simulink model "ap_12B_cocoSim_pp"  (Simulink 8.5)
settings: Solver=ode3  StartTime=0.0  StopTime=100  FixedStep=Ts  RelTol=1e-3
undefined symbols (not defined in the file): beaver_b, beaver_c, beaver_mass, beaver_S, Cl0, Cl_alpha2_dpt, Cl_beta, Cl_da, Cl_da_alpha, Cl_dr, Cl_p, Cl_r, Cm0, Cm_alpha, Cm_alpha2, Cm_beta2, Cm_de, Cm_df, Cm_dpt, Cm_q, Cm_r, Cn0, Cn_beta, Cn_beta3, Cn_da, Cn_dpt3, Cn_dr, Cn_p, Cn_q, Cn_r, Cx0, Cx_alpha, Cx_alpha2, Cx_alpha3, Cx_df, Cx_df_alpha, Cx_dpt, Cx_dpt2_alpha, Cx_dr, Cx_q, Cy0, Cy_beta, Cy_da, Cy_dr, Cy_dr_alpha, Cy_p, Cy_r, Cz0, Cz_alpha, Cz_alpha3, Cz_de, Cz_de_beta, Cz_df, Cz_df_alpha, Cz_dpt, Cz_q, d2r, fin_act_1, fin_act_2, fin_act_3 ... (+23)
libraries: simulink x12, aerolibtransform2 x9, aerolibutil x7, aerolibasang x7, aerolibadynsys x3, aerolib6dofsys x2, aerolib6dof2 x1
(part 2 of 3)

== system ap_12B_cocoSim_pp/Autopilot/Roll_Autopilot/Roll Reference ==
  note: Roll Reference
  Phi : Inport  RequirementInfo={'other' 'do178b_autopilot_requirements.docx' '@Simulink_requirement_item_3' 'true' '1.3. Roll Hold Reference' '' } %GIDa_7be110a1_1244_43c5_a751_2715cb6886db
  AP eng : Inport  RequirementInfo={'other' 'do178b_autopilot_requirements.docx' '@Simulink_requirement_item_3' 'true' '1.3. Roll Hold Reference' '' } %GIDa_7321b38e_2b45_4502_bb86_556b63306af0  Port=2
  Turn Knob : Inport  RequirementInfo={'other' 'do178b_autopilot_requirements.docx' '@Simulink_requirement_item_3' 'true' '1.3. Roll Hold Reference' '' } %GIDa_fd11246b_c871_46a3_9662_7459fa475b84  Port=3
  Abs : Abs  RequirementInfo={'other' 'do178b_autopilot_requirements.docx' '@Simulink_requirement_item_3' 'true' '1.3. Roll Hold Reference' '' } %GIDa_7c5a478a_1c5c_492b_92bb_3b8cbe69ec92
  Not engaged : Logic  RequirementInfo={'other' 'do178b_autopilot_requirements.docx' '@Simulink_requirement_item_3' 'true' '1.3. Roll Hold Reference' '' } %GIDa_f8de7ddf_282c_452d_ba2b_b5d1c603b30d  Operator=NOT  IconShape=distinctive  AllPortsSameDT=off  OutDataTypeStr=boolean
  Ref Threshold : RelationalOperator  RequirementInfo={'other' 'do178b_autopilot_requirements.docx' '@Simulink_requirement_item_3' 'true' '1.3. Roll Hold Reference' '' } %GIDa_5bcc0fb3_b840_4e41_b948_77b94adee73e  OutDataTypeStr=boolean  InputSameDT=on
  Ref Threshold1 : RelationalOperator  RequirementInfo={'other' 'do178b_autopilot_requirements.docx' '@Simulink_requirement_item_3' 'true' '1.3. Roll Hold Reference' '' } %GIDa_b386a317_4628_4582_ad41_ffeb1b32dfb2  Operator=<=  OutDataTypeStr=boolean  InputSameDT=on
  TK Threshold : RelationalOperator  RequirementInfo={'other' 'do178b_autopilot_requirements.docx' '@Simulink_requirement_item_3' 'true' '1.3. Roll Hold Reference' '' } %GIDa_e8f6e4ba_d398_47e9_910c_6097861fe37d  Operator=<  OutDataTypeStr=boolean  InputSameDT=on
  TK switch : Switch  RequirementInfo={'other' 'do178b_autopilot_requirements.docx' '@Simulink_requirement_item_3' 'true' '1.3. Roll Hold Reference' '' } %GIDa_ffde3420_eaf1_4246_b6be_15fcaa55a732  Criteria=u2 ~= 0
  latch : Subsystem
  minus six : Constant  RequirementInfo={'other' 'do178b_autopilot_requirements.docx' '@Simulink_requirement_item_3' 'true' '1.3. Roll Hold Reference' '' } %GIDa_48756242_1906_4ef4_8b8e_98d44b831f1a  Value=-6
  or : Logic  RequirementInfo={'other' 'do178b_autopilot_requirements.docx' '@Simulink_requirement_item_3' 'true' '1.3. Roll Hold Reference' '' } %GIDa_e1ded3c2_ef34_4c5e_a646_1c97eb11feb3  Operator=OR  IconShape=distinctive  OutDataTypeStr=boolean
  ref switch : Switch  RequirementInfo={'other' 'do178b_autopilot_requirements.docx' '@Simulink_requirement_item_3' 'true' '1.3. Roll Hold Reference' '' } %GIDa_b3ccb91c_c36a_487a_a60d_dccfbea1bfea  Criteria=u2 ~= 0
  six : Constant  RequirementInfo={'other' 'do178b_autopilot_requirements.docx' '@Simulink_requirement_item_3' 'true' '1.3. Roll Hold Reference' '' } %GIDa_126d714f_9b47_471a_b875_8464e4535534  Value=6
  three : Constant  RequirementInfo={'other' 'do178b_autopilot_requirements.docx' '@Simulink_requirement_item_3' 'true' '1.3. Roll Hold Reference' '' } %GIDa_1a721058_8682_40e6_baec_2d04b535a447  Value=3  OutDataTypeStr=double
  zero : Constant  RequirementInfo={'other' 'do178b_autopilot_requirements.docx' '@Simulink_requirement_item_3' 'true' '1.3. Roll Hold Reference' '' } %GIDa_1aabe46b_3def_4f63_9213_51ab779e4755  Value=0
  Phi Ref : Outport  RequirementInfo={'other' 'do178b_autopilot_requirements.docx' '@Simulink_requirement_item_3' 'true' '1.3. Roll Hold Reference' '' } %GIDa_b84f1043_d8b5_4dd2_9707_41139a24d3a9
  wires:
  minus six/1 -> Ref Threshold1/2
  Ref Threshold1/1 -> or/2
  Ref Threshold/1 -> or/1
  or/1 -> ref switch/2
  zero/1 -> ref switch/3
  six/1 -> Ref Threshold/2
  TK switch/1 -> Phi Ref/1
  AP eng/1 -> Not engaged/1
  Phi/1 -> Ref Threshold1/1, Ref Threshold/1, ref switch/1
  Abs/1 -> TK Threshold/1
  three/1 -> TK Threshold/2
  Turn Knob/1 -> Abs/1, TK switch/3
  TK Threshold/1 -> TK switch/2
  latch/1(y) -> TK switch/1
  ref switch/1 -> latch/1(u)
  Not engaged/1 -> latch/2(E)

== system ap_12B_cocoSim_pp/Autopilot/Yaw_damper/Basic Yaw Damper ==
  note: Basic Yaw Damper
  "Phi " : Inport
  R : Inport  Port=2
  TAS : Inport  Port=3
  Constant : Constant  Value=100
  MinMax : MinMax  Function=max  Inputs=2
  Model Info : simulink/Model-Wide Utilities/Model Info  BlockCM=None  Frame=on  DisplayStringWithTags=|  HorizontalTextAlignment=Left  LeftAlignmentValue=0.02  SourceBlockDiagram=ap_12B_cocoSim_pp  TagMaxNumber=20
      | Yaw Damper
      | Author: %<LastModifiedBy>
      | Date: %<LastModificationDate>
      | Model Version: %<ModelVersion>
  Product : Product  Inputs=*/  RndMeth=Zero
  Rate Gain : Gain  Gain=1.0
  Rud Limit : Saturate  UpperLimit=25  LowerLimit=-25
      settings: AttributesFormatString=%<LowerLimit> to %<UpperLimit> (deg)
  Sum1 : Sum  Inputs=|+-
  gravity : Gain  Gain=32.2
  sin : Trigonometry
  Rud Cmd : Outport
  wires:
  R/1 -> Sum1/2
  Sum1/1 -> Rate Gain/1  "yawRate"
  Rud Limit/1 -> Rud Cmd/1
  Rate Gain/1 -> Rud Limit/1
  "Phi "/1 -> sin/1
  sin/1 -> gravity/1
  Product/1 -> Sum1/1
  gravity/1 -> Product/1
  MinMax/1 -> Product/2
  TAS/1 -> MinMax/1
  Constant/1 -> MinMax/2

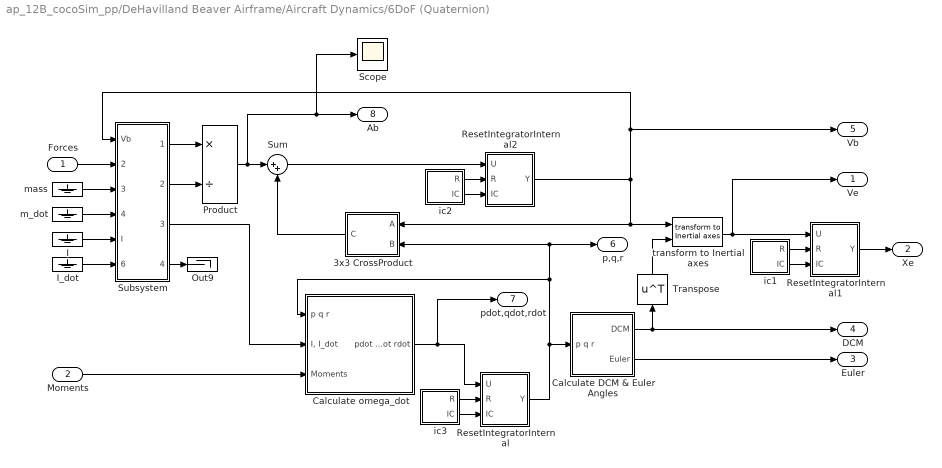
== system ap_12B_cocoSim_pp/DeHavilland Beaver Airframe/Aircraft Dynamics/6DoF (Quaternion) ==
  Forces : Inport
  Moments : Inport  Port=2
  3x3 CrossProduct : Subsystem
  Calculate DCM & Euler Angles : Subsystem
  Calculate omega_dot : Subsystem
  I : Ground
  I_dot : Ground
  Out9 : Terminator
  Product : Product  Inputs=*/  SaturateOnIntegerOverflow=on  OutDataTypeStr=Inherit: Same as first input
  ResetIntegratorInternal : Subsystem
  ResetIntegratorInternal1 : Subsystem
  ResetIntegratorInternal2 : Subsystem
  Scope : Scope
      settings: SaveName=ScopeData4
  Subsystem : Subsystem
  Sum : Sum  Inputs=|++  SaturateOnIntegerOverflow=on
  Transpose : Math  Operator=transpose  SaturateOnIntegerOverflow=on
  ic1 : Subsystem
  ic2 : Subsystem
  ic3 : Subsystem
  m_dot : Ground
  mass : Ground
  "transform to Inertial axes " : aerolib6dof2/6DoF (Euler Angles)/transform to Inertial axes   SystemSampleTime=-1
  Ve : Outport
  Xe : Outport  Port=2
  Euler : Outport  Port=3
  DCM : Outport  Port=4
  Vb : Outport  Port=5
  p,q,r : Outport  Port=6
  pdot,qdot,rdot : Outport  Port=7
  Ab : Outport  Port=8
  wires:
  Subsystem/1("forces ") -> Product/1
  I_dot/1 -> Subsystem/6(I_dot)
  I/1 -> Subsystem/5(I)
  Calculate omega_dot/1(pdot qdot rdot) -> pdot,qdot,rdot/1, ResetIntegratorInternal/1(U)
  Subsystem/4(Out9) -> Out9/1
  m_dot/1 -> Subsystem/4(m_dot)
  Subsystem/2(mass) -> Product/2
  mass/1 -> Subsystem/3("mass ")
  Transpose/1 -> "transform to Inertial axes "/2
  Calculate DCM & Euler Angles/1(DCM) -> DCM/1, Transpose/1
  Product/1 -> Scope/1, Ab/1, Sum/1
  Forces/1 -> Subsystem/2(forces)
  Moments/1 -> Calculate omega_dot/3(Moments)
  ResetIntegratorInternal1/1(Y) -> Xe/1
  Sum/1 -> ResetIntegratorInternal2/1(U)
  3x3 CrossProduct/1(C) -> Sum/2
  Calculate DCM & Euler Angles/2(Euler) -> Euler/1
  Subsystem/3("inertia, 0") -> Calculate omega_dot/2("I, I_dot")
  "transform to Inertial axes "/1 -> ResetIntegratorInternal1/1(U), Ve/1
  ResetIntegratorInternal/1(Y) -> Calculate DCM & Euler Angles/1(p q r), 3x3 CrossProduct/2(B), p,q,r/1, Calculate omega_dot/1(p q r)
  ic3/1(R) -> ResetIntegratorInternal/2(R)
  ic3/2(IC) -> ResetIntegratorInternal/3(IC)
  ic1/1(R) -> ResetIntegratorInternal1/2(R)
  ic1/2(IC) -> ResetIntegratorInternal1/3(IC)
  ic2/1(R) -> ResetIntegratorInternal2/2(R)
  ic2/2(IC) -> ResetIntegratorInternal2/3(IC)
  ResetIntegratorInternal2/1(Y) -> Subsystem/1(Vb), Vb/1, 3x3 CrossProduct/1(A), "transform to Inertial axes "/1

== system ap_12B_cocoSim_pp/DeHavilland Beaver Airframe/Aircraft Dynamics/Total Forces  and Moments ==
  EnvirBus : Inport
  Pilot : Inport  Port=2
  DCM : Inport  Port=3
  FltParams : Inport  Port=4
  Actuators : Subsystem
  Aerodynamics : Subsystem
  Bus Selector4 : BusSelector  OutputSignals=rho,g
  "Engine " : Subsystem
  Forces and Moments : Subsystem
  "Gravity " : Subsystem
  "Pilot " : InportShadow  Port=2
  Sum : Sum  Inputs=|++  SaturateOnIntegerOverflow=on  InputSameDT=on  OutDataTypeStr=Inherit: Same as first input
  Total Force : Outport
  Total Moment : Outport  Port=2
  wires:
  Forces and Moments/1(XYZ) -> Sum/1
  "Engine "/1(Engine Coefficients) -> Forces and Moments/3(Engine Coefficients)
  "Gravity "/1(Fgrav) -> Sum/2
  Aerodynamics/1(Aero Coefficients) -> Forces and Moments/1(Aero Coefficients)
  Pilot/1 -> Actuators/1(Pilot)
  Bus Selector4/1 -> "Engine "/3(rho)  "<rho>"
  DCM/1 -> "Gravity "/2(DCM)
  Bus Selector4/2 -> "Gravity "/1(g)  "<g>"
  Sum/1 -> Total Force/1  "Ftot"
  Forces and Moments/2(LMN) -> Total Moment/1  "Mtot"
  "Pilot "/1 -> "Engine "/2(Pilot)
  FltParams/1 -> Forces and Moments/2(Fltparams), "Engine "/1(Fltparams), Aerodynamics/2(FltParams)
  Actuators/1(uaero-out) -> Aerodynamics/1(Uaero)
  EnvirBus/1 -> Bus Selector4/1

== system ap_12B_cocoSim_pp/DeHavilland Beaver Airframe/Calculate Parameters/ Incidence, Sideslip,  & Airspeed ==
  Vb : Inport
  Airspeed : Sqrt  AlgorithmType=Newton-Raphson  SaturateOnIntegerOverflow=on
  Incidence : Trigonometry  Operator=atan2
  Product : Product  Inputs=*/  SaturateOnIntegerOverflow=on  OutDataTypeStr=Inherit: Same as first input
  Sideslip : Trigonometry  Operator=asin
  Subsystem : aerolibasang/Incidence, Sideslip, & Airspeed/Subsystem
  Subsystem1 : aerolibasang/Incidence, Sideslip, & Airspeed/Subsystem1
  dot : aerolibasang/Incidence, Sideslip, & Airspeed/dot
  Alpha : Outport  InitialOutput=0
  Beta : Outport  Port=2  InitialOutput=0
  V : Outport  Port=3  InitialOutput=0
  wires:
  Sideslip/1 -> Beta/1
  Subsystem1/1 -> Product/1
  Product/1 -> Sideslip/1
  Subsystem/1 -> Incidence/1
  Subsystem/2 -> Incidence/2
  dot/1 -> Airspeed/1
  Airspeed/1 -> V/1, Product/2
  Incidence/1 -> Alpha/1
  Vb/1 -> Subsystem/1, dot/1, Subsystem1/1

== system ap_12B_cocoSim_pp/DeHavilland Beaver Airframe/Calculate Parameters/Dynamic Pressure ==
  Velocity : Inport
  Air Density : Inport  Port=2
  1/2rhoV^2 : Gain  Gain=0.5  SaturateOnIntegerOverflow=on  OutDataTypeStr=Inherit: Same as input  ParamDataTypeStr=Inherit: Same as input
  Product2 : Product  SaturateOnIntegerOverflow=on  InputSameDT=on  OutDataTypeStr=Inherit: Same as first input
  dot : aerolibasang/Dynamic Pressure/dot
  qbar : Outport  InitialOutput=0
  wires:
  1/2rhoV^2/1 -> qbar/1
  Air Density/1 -> Product2/2
  dot/1 -> Product2/1
  Product2/1 -> 1/2rhoV^2/1
  Velocity/1 -> dot/1

== system ap_12B_cocoSim_pp/Sensors/Air Data Sensor/ Incidence, Sideslip,  & Airspeed ==
  Vb : Inport
  Airspeed : Sqrt  AlgorithmType=Newton-Raphson  SaturateOnIntegerOverflow=on
  Gain : Gain  Gain=180/pi
  Gain1 : Gain  Gain=180/pi
  Incidence : Trigonometry  Operator=atan2
  Product : Product  Inputs=*/  SaturateOnIntegerOverflow=on  OutDataTypeStr=Inherit: Same as first input
  Scope : Scope
      settings: SaveName=ScopeData24
  Scope1 : Scope
      settings: SaveName=ScopeData25
  Sideslip : Trigonometry  Operator=asin
  Subsystem : aerolibasang/Incidence, Sideslip, & Airspeed/Subsystem
  Subsystem1 : aerolibasang/Incidence, Sideslip, & Airspeed/Subsystem1
  dot : aerolibasang/Incidence, Sideslip, & Airspeed/dot
  Alpha : Outport  InitialOutput=0
  Beta : Outport  Port=2  InitialOutput=0
  V : Outport  Port=3  InitialOutput=0
  wires:
  Sideslip/1 -> Gain1/1, Beta/1
  Subsystem1/1 -> Product/1
  Product/1 -> Sideslip/1
  Subsystem/1 -> Incidence/1
  Subsystem/2 -> Incidence/2
  dot/1 -> Airspeed/1
  Airspeed/1 -> V/1, Product/2
  Incidence/1 -> Gain/1, Alpha/1
  Vb/1 -> Subsystem/1, dot/1, Subsystem1/1
  Gain/1 -> Scope/1
  Gain1/1 -> Scope1/1

== system ap_12B_cocoSim_pp/Sensors/Air Data Sensor/ic1 ==
  u : Inport
  ic : Inport  Port=2
  Constant : Constant
  Switch : Switch  Criteria=u2 ~= 0
  Unit Delay : UnitDelay  SampleTime=-1
  y : Outport
  wires:
  Switch/1 -> y/1
  u/1 -> Switch/1
  ic/1 -> Switch/3
  Constant/1 -> Unit Delay/1
  Unit Delay/1 -> Switch/2

== system ap_12B_cocoSim_pp/Sensors/Air Data Sensor/ic2 ==
  u : Inport
  ic : Inport  Port=2
  Constant : Constant
  Switch : Switch  Criteria=u2 ~= 0
  Unit Delay : UnitDelay  SampleTime=-1
  y : Outport
  wires:
  ic/1 -> Switch/3
  u/1 -> Switch/1
  Switch/1 -> y/1
  Constant/1 -> Unit Delay/1
  Unit Delay/1 -> Switch/2

== system ap_12B_cocoSim_pp/Sensors/Air Data Sensor/ic3 ==
  u : Inport
  ic : Inport  Port=2
  Constant1 : Constant
  Switch : Switch  Criteria=u2 ~= 0
  Unit Delay1 : UnitDelay  SampleTime=-1
  y : Outport
  wires:
  ic/1 -> Switch/3
  u/1 -> Switch/1
  Switch/1 -> y/1
  Constant1/1 -> Unit Delay1/1
  Unit Delay1/1 -> Switch/2

== system ap_12B_cocoSim_pp/Sensors/Inertial Data Sensor/ic ==
  u : Inport
  ic : Inport  Port=2
  Constant : Constant
  Switch : Switch  Criteria=u2 ~= 0
  Unit Delay : UnitDelay  SampleTime=-1
  y : Outport
  wires:
  Switch/1 -> y/1
  u/1 -> Switch/1
  ic/1 -> Switch/3
  Constant/1 -> Unit Delay/1
  Unit Delay/1 -> Switch/2

== system ap_12B_cocoSim_pp/Sensors/Inertial Data Sensor/ic1 ==
  u : Inport
  ic : Inport  Port=2
  Constant : Constant
  Switch : Switch  Criteria=u2 ~= 0
  Unit Delay : UnitDelay  SampleTime=-1
  y : Outport
  wires:
  ic/1 -> Switch/3
  u/1 -> Switch/1
  Switch/1 -> y/1
  Constant/1 -> Unit Delay/1
  Unit Delay/1 -> Switch/2

== system ap_12B_cocoSim_pp/Sensors/Inertial Data Sensor/ic2 ==
  u : Inport
  ic : Inport  Port=2
  Constant : Constant
  Switch : Switch  Criteria=u2 ~= 0
  Unit Delay : UnitDelay  SampleTime=-1
  y : Outport
  wires:
  Switch/1 -> y/1
  u/1 -> Switch/1
  ic/1 -> Switch/3
  Constant/1 -> Unit Delay/1
  Unit Delay/1 -> Switch/2

== system ap_12B_cocoSim_pp/Sensors/Inertial Data Sensor/ic3 ==
  u : Inport
  ic : Inport  Port=2
  Constant : Constant
  Switch : Switch  Criteria=u2 ~= 0
  Unit Delay : UnitDelay  SampleTime=-1
  y : Outport
  wires:
  ic/1 -> Switch/3
  u/1 -> Switch/1
  Switch/1 -> y/1
  Constant/1 -> Unit Delay/1
  Unit Delay/1 -> Switch/2

== system ap_12B_cocoSim_pp/Signal Conditioning/RPM2ManifoldPressure_pp/Interpolate1 ==
  InportIn : Inport
  InportIdx1 : Inport  Port=2
  InportIdx2 : Inport  Port=3
  InportData1 : Inport  Port=4
  InportData2 : Inport  Port=5
  Interpolate : Product  Inputs=*/*  SaturateOnIntegerOverflow=on  RndMeth=Zero  InputSameDT=on  OutDataTypeStr=Inherit: Same as first input
  Sum1 : Sum  Inputs=+-  SaturateOnIntegerOverflow=on  InputSameDT=on  OutDataTypeStr=Inherit: Same as first input
  Sum2 : Sum  Inputs=-+  SaturateOnIntegerOverflow=on  InputSameDT=on  OutDataTypeStr=Inherit: Same as first input
  Sum3 : Sum  Inputs=-+  SaturateOnIntegerOverflow=on  InputSameDT=on  OutDataTypeStr=Inherit: Same as first input
  Sum4 : Sum  SaturateOnIntegerOverflow=on  InputSameDT=on  OutDataTypeStr=Inherit: Same as first input
  Out : Outport
  wires:
  InportIn/1 -> Sum1/1
  InportIdx1/1 -> Sum1/2, Sum2/1
  InportIdx2/1 -> Sum2/2
  InportData1/1 -> Sum3/1, Sum4/2
  InportData2/1 -> Sum3/2
  Sum1/1 -> Interpolate/1
  Sum2/1 -> Interpolate/2
  Sum3/1 -> Interpolate/3
  Interpolate/1 -> Sum4/1
  Sum4/1 -> Out/1

== system ap_12B_cocoSim_pp/Signal Conditioning/RPM2ManifoldPressure_pp/Interpolate2 ==
  InportIn : Inport
  InportIdx1 : Inport  Port=2
  InportIdx2 : Inport  Port=3
  InportData1 : Inport  Port=4
  InportData2 : Inport  Port=5
  Interpolate : Product  Inputs=*/*  SaturateOnIntegerOverflow=on  RndMeth=Zero  InputSameDT=on  OutDataTypeStr=Inherit: Same as first input
  Sum1 : Sum  Inputs=+-  SaturateOnIntegerOverflow=on  InputSameDT=on  OutDataTypeStr=Inherit: Same as first input
  Sum2 : Sum  Inputs=-+  SaturateOnIntegerOverflow=on  InputSameDT=on  OutDataTypeStr=Inherit: Same as first input
  Sum3 : Sum  Inputs=-+  SaturateOnIntegerOverflow=on  InputSameDT=on  OutDataTypeStr=Inherit: Same as first input
  Sum4 : Sum  SaturateOnIntegerOverflow=on  InputSameDT=on  OutDataTypeStr=Inherit: Same as first input
  Out : Outport
  wires:
  InportIn/1 -> Sum1/1
  InportIdx1/1 -> Sum1/2, Sum2/1
  InportIdx2/1 -> Sum2/2
  InportData1/1 -> Sum3/1, Sum4/2
  InportData2/1 -> Sum3/2
  Sum1/1 -> Interpolate/1
  Sum2/1 -> Interpolate/2
  Sum3/1 -> Interpolate/3
  Interpolate/1 -> Sum4/1
  Sum4/1 -> Out/1

== system ap_12B_cocoSim_pp/Signal Conditioning/Throttle2RPM_pp/Interpolate1 ==
  InportIn : Inport
  InportIdx1 : Inport  Port=2
  InportIdx2 : Inport  Port=3
  InportData1 : Inport  Port=4
  InportData2 : Inport  Port=5
  Interpolate : Product  Inputs=*/*  SaturateOnIntegerOverflow=on  RndMeth=Zero  InputSameDT=on  OutDataTypeStr=Inherit: Same as first input
  Sum1 : Sum  Inputs=+-  SaturateOnIntegerOverflow=on  InputSameDT=on  OutDataTypeStr=Inherit: Same as first input
  Sum2 : Sum  Inputs=-+  SaturateOnIntegerOverflow=on  InputSameDT=on  OutDataTypeStr=Inherit: Same as first input
  Sum3 : Sum  Inputs=-+  SaturateOnIntegerOverflow=on  InputSameDT=on  OutDataTypeStr=Inherit: Same as first input
  Sum4 : Sum  SaturateOnIntegerOverflow=on  InputSameDT=on  OutDataTypeStr=Inherit: Same as first input
  Out : Outport
  wires:
  InportIn/1 -> Sum1/1
  InportIdx1/1 -> Sum1/2, Sum2/1
  InportIdx2/1 -> Sum2/2
  InportData1/1 -> Sum3/1, Sum4/2
  InportData2/1 -> Sum3/2
  Sum1/1 -> Interpolate/1
  Sum2/1 -> Interpolate/2
  Sum3/1 -> Interpolate/3
  Interpolate/1 -> Sum4/1
  Sum4/1 -> Out/1

== system ap_12B_cocoSim_pp/Signal Conditioning/Throttle2RPM_pp/Interpolate2 ==
  InportIn : Inport
  InportIdx1 : Inport  Port=2
  InportIdx2 : Inport  Port=3
  InportData1 : Inport  Port=4
  InportData2 : Inport  Port=5
  Interpolate : Product  Inputs=*/*  SaturateOnIntegerOverflow=on  RndMeth=Zero  InputSameDT=on  OutDataTypeStr=Inherit: Same as first input
  Sum1 : Sum  Inputs=+-  SaturateOnIntegerOverflow=on  InputSameDT=on  OutDataTypeStr=Inherit: Same as first input
  Sum2 : Sum  Inputs=-+  SaturateOnIntegerOverflow=on  InputSameDT=on  OutDataTypeStr=Inherit: Same as first input
  Sum3 : Sum  Inputs=-+  SaturateOnIntegerOverflow=on  InputSameDT=on  OutDataTypeStr=Inherit: Same as first input
  Sum4 : Sum  SaturateOnIntegerOverflow=on  InputSameDT=on  OutDataTypeStr=Inherit: Same as first input
  Out : Outport
  wires:
  InportIn/1 -> Sum1/1
  InportIdx1/1 -> Sum1/2, Sum2/1
  InportIdx2/1 -> Sum2/2
  InportData1/1 -> Sum3/1, Sum4/2
  InportData2/1 -> Sum3/2
  Sum1/1 -> Interpolate/1
  Sum2/1 -> Interpolate/2
  Sum3/1 -> Interpolate/3
  Interpolate/1 -> Sum4/1
  Sum4/1 -> Out/1

== system ap_12B_cocoSim_pp/Signal Conditioning/Throttle2RPM_pp/Interpolate3 ==
  InportIn : Inport
  InportIdx1 : Inport  Port=2
  InportIdx2 : Inport  Port=3
  InportData1 : Inport  Port=4
  InportData2 : Inport  Port=5
  Interpolate : Product  Inputs=*/*  SaturateOnIntegerOverflow=on  RndMeth=Zero  InputSameDT=on  OutDataTypeStr=Inherit: Same as first input
  Sum1 : Sum  Inputs=+-  SaturateOnIntegerOverflow=on  InputSameDT=on  OutDataTypeStr=Inherit: Same as first input
  Sum2 : Sum  Inputs=-+  SaturateOnIntegerOverflow=on  InputSameDT=on  OutDataTypeStr=Inherit: Same as first input
  Sum3 : Sum  Inputs=-+  SaturateOnIntegerOverflow=on  InputSameDT=on  OutDataTypeStr=Inherit: Same as first input
  Sum4 : Sum  SaturateOnIntegerOverflow=on  InputSameDT=on  OutDataTypeStr=Inherit: Same as first input
  Out : Outport
  wires:
  InportIn/1 -> Sum1/1
  InportIdx1/1 -> Sum1/2, Sum2/1
  InportIdx2/1 -> Sum2/2
  InportData1/1 -> Sum3/1, Sum4/2
  InportData2/1 -> Sum3/2
  Sum1/1 -> Interpolate/1
  Sum2/1 -> Interpolate/2
  Sum3/1 -> Interpolate/3
  Interpolate/1 -> Sum4/1
  Sum4/1 -> Out/1

== system ap_12B_cocoSim_pp/Signal Conditioning/Throttle2RPM_pp/Interpolate4 ==
  InportIn : Inport
  InportIdx1 : Inport  Port=2
  InportIdx2 : Inport  Port=3
  InportData1 : Inport  Port=4
  InportData2 : Inport  Port=5
  Interpolate : Product  Inputs=*/*  SaturateOnIntegerOverflow=on  RndMeth=Zero  InputSameDT=on  OutDataTypeStr=Inherit: Same as first input
  Sum1 : Sum  Inputs=+-  SaturateOnIntegerOverflow=on  InputSameDT=on  OutDataTypeStr=Inherit: Same as first input
  Sum2 : Sum  Inputs=-+  SaturateOnIntegerOverflow=on  InputSameDT=on  OutDataTypeStr=Inherit: Same as first input
  Sum3 : Sum  Inputs=-+  SaturateOnIntegerOverflow=on  InputSameDT=on  OutDataTypeStr=Inherit: Same as first input
  Sum4 : Sum  SaturateOnIntegerOverflow=on  InputSameDT=on  OutDataTypeStr=Inherit: Same as first input
  Out : Outport
  wires:
  InportIn/1 -> Sum1/1
  InportIdx1/1 -> Sum1/2, Sum2/1
  InportIdx2/1 -> Sum2/2
  InportData1/1 -> Sum3/1, Sum4/2
  InportData2/1 -> Sum3/2
  Sum1/1 -> Interpolate/1
  Sum2/1 -> Interpolate/2
  Sum3/1 -> Interpolate/3
  Interpolate/1 -> Sum4/1
  Sum4/1 -> Out/1

== system ap_12B_cocoSim_pp/Signal Conditioning/Throttle2RPM_pp/Interpolate5 ==
  InportIn : Inport
  InportIdx1 : Inport  Port=2
  InportIdx2 : Inport  Port=3
  InportData1 : Inport  Port=4
  InportData2 : Inport  Port=5
  Interpolate : Product  Inputs=*/*  SaturateOnIntegerOverflow=on  RndMeth=Zero  InputSameDT=on  OutDataTypeStr=Inherit: Same as first input
  Sum1 : Sum  Inputs=+-  SaturateOnIntegerOverflow=on  InputSameDT=on  OutDataTypeStr=Inherit: Same as first input
  Sum2 : Sum  Inputs=-+  SaturateOnIntegerOverflow=on  InputSameDT=on  OutDataTypeStr=Inherit: Same as first input
  Sum3 : Sum  Inputs=-+  SaturateOnIntegerOverflow=on  InputSameDT=on  OutDataTypeStr=Inherit: Same as first input
  Sum4 : Sum  SaturateOnIntegerOverflow=on  InputSameDT=on  OutDataTypeStr=Inherit: Same as first input
  Out : Outport
  wires:
  InportIn/1 -> Sum1/1
  InportIdx1/1 -> Sum1/2, Sum2/1
  InportIdx2/1 -> Sum2/2
  InportData1/1 -> Sum3/1, Sum4/2
  InportData2/1 -> Sum3/2
  Sum1/1 -> Interpolate/1
  Sum2/1 -> Interpolate/2
  Sum3/1 -> Interpolate/3
  Interpolate/1 -> Sum4/1
  Sum4/1 -> Out/1

== system ap_12B_cocoSim_pp/Signal Conditioning/Throttle2RPM_pp/Interpolate6 ==
  InportIn : Inport
  InportIdx1 : Inport  Port=2
  InportIdx2 : Inport  Port=3
  InportData1 : Inport  Port=4
  InportData2 : Inport  Port=5
  Interpolate : Product  Inputs=*/*  SaturateOnIntegerOverflow=on  RndMeth=Zero  InputSameDT=on  OutDataTypeStr=Inherit: Same as first input
  Sum1 : Sum  Inputs=+-  SaturateOnIntegerOverflow=on  InputSameDT=on  OutDataTypeStr=Inherit: Same as first input
  Sum2 : Sum  Inputs=-+  SaturateOnIntegerOverflow=on  InputSameDT=on  OutDataTypeStr=Inherit: Same as first input
  Sum3 : Sum  Inputs=-+  SaturateOnIntegerOverflow=on  InputSameDT=on  OutDataTypeStr=Inherit: Same as first input
  Sum4 : Sum  SaturateOnIntegerOverflow=on  InputSameDT=on  OutDataTypeStr=Inherit: Same as first input
  Out : Outport
  wires:
  InportIn/1 -> Sum1/1
  InportIdx1/1 -> Sum1/2, Sum2/1
  InportIdx2/1 -> Sum2/2
  InportData1/1 -> Sum3/1, Sum4/2
  InportData2/1 -> Sum3/2
  Sum1/1 -> Interpolate/1
  Sum2/1 -> Interpolate/2
  Sum3/1 -> Interpolate/3
  Interpolate/1 -> Sum4/1
  Sum4/1 -> Out/1

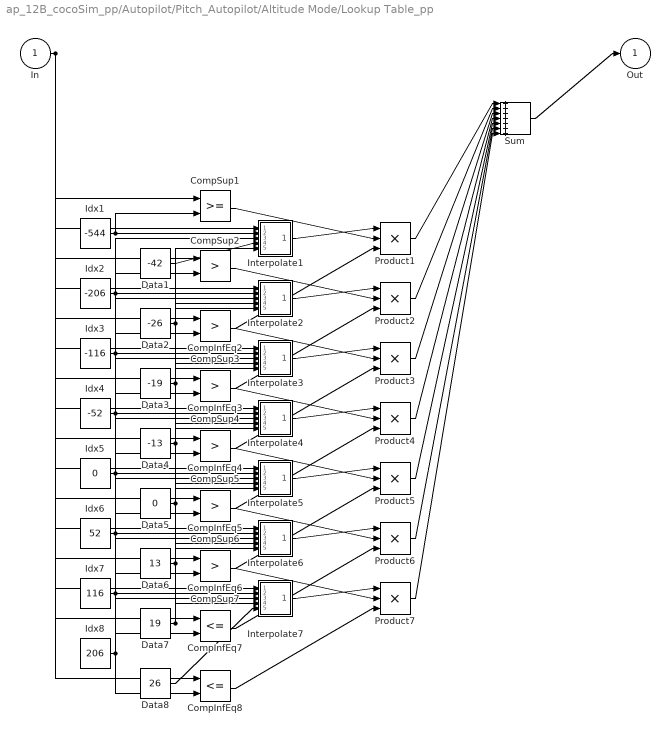
== system ap_12B_cocoSim_pp/Autopilot/Pitch_Autopilot/Altitude Mode/Lookup Table_pp ==
  In : Inport
  CompInfEq{2..8} (7 alike) : RelationalOperator  Operator=<=  InputSameDT=on
  CompSup1 : RelationalOperator  InputSameDT=on
  CompSup{2..7} (6 alike) : RelationalOperator  Operator=>  InputSameDT=on
  Data1 : Constant  Value=-42
  Data2 : Constant  Value=-26
  Data3 : Constant  Value=-19
  Data4 : Constant  Value=-13
  Data5 : Constant  Value=0
  Data6 : Constant  Value=13
  Data7 : Constant  Value=19
  Data8 : Constant  Value=26
  Idx1 : Constant  Value=-544
  Idx2 : Constant  Value=-206
  Idx3 : Constant  Value=-116
  Idx4 : Constant  Value=-52
  Idx5 : Constant  Value=0
  Idx6 : Constant  Value=52
  Idx7 : Constant  Value=116
  Idx8 : Constant  Value=206
  Interpolate1 : Subsystem
  Interpolate2 : Subsystem
  Interpolate3 : Subsystem
  Interpolate4 : Subsystem
  Interpolate5 : Subsystem
  Interpolate6 : Subsystem
  Interpolate7 : Subsystem
  Product{1..7} (7 alike) : Product  Inputs=***  SaturateOnIntegerOverflow=on  RndMeth=Zero  OutDataTypeStr=Inherit: Same as first input
  Sum : Sum  Inputs=+++++++  SaturateOnIntegerOverflow=on  InputSameDT=on  OutDataTypeStr=Inherit: Same as first input
  Out : Outport
  wires:
  In/1 -> Interpolate1/1(InportIn), CompSup1/1, Interpolate2/1(InportIn), CompSup2/1, CompInfEq2/1, Interpolate3/1(InportIn), CompSup3/1, CompInfEq3/1, Interpolate4/1(InportIn), CompSup4/1, CompInfEq4/1, Interpolate5/1(InportIn), CompSup5/1, CompInfEq5/1, Interpolate6/1(InportIn), CompSup6/1, CompInfEq6/1, Interpolate7/1(InportIn), CompSup7/1, CompInfEq7/1, CompInfEq8/1
  Idx1/1 -> Interpolate1/2(InportIdx1), CompSup1/2
  Data1/1 -> Interpolate1/4(InportData1)
  Interpolate1/1(Out) -> Product1/1
  CompSup1/1 -> Product1/2
  CompInfEq2/1 -> Product1/3
  Product1/1 -> Sum/1
  Idx2/1 -> Interpolate2/2(InportIdx1), CompSup2/2, Interpolate1/3(InportIdx2), CompInfEq2/2
  Data2/1 -> Interpolate2/4(InportData1), Interpolate1/5(InportData2)
  Interpolate2/1(Out) -> Product2/1
  CompSup2/1 -> Product2/2
  CompInfEq3/1 -> Product2/3
  Product2/1 -> Sum/2
  Idx3/1 -> Interpolate3/2(InportIdx1), CompSup3/2, Interpolate2/3(InportIdx2), CompInfEq3/2
  Data3/1 -> Interpolate3/4(InportData1), Interpolate2/5(InportData2)
  Interpolate3/1(Out) -> Product3/1
  CompSup3/1 -> Product3/2
  CompInfEq4/1 -> Product3/3
  Product3/1 -> Sum/3
  Idx4/1 -> Interpolate4/2(InportIdx1), CompSup4/2, Interpolate3/3(InportIdx2), CompInfEq4/2
  Data4/1 -> Interpolate4/4(InportData1), Interpolate3/5(InportData2)
  Interpolate4/1(Out) -> Product4/1
  CompSup4/1 -> Product4/2
  CompInfEq5/1 -> Product4/3
  Product4/1 -> Sum/4
  Idx5/1 -> Interpolate5/2(InportIdx1), CompSup5/2, Interpolate4/3(InportIdx2), CompInfEq5/2
  Data5/1 -> Interpolate5/4(InportData1), Interpolate4/5(InportData2)
  Interpolate5/1(Out) -> Product5/1
  CompSup5/1 -> Product5/2
  CompInfEq6/1 -> Product5/3
  Product5/1 -> Sum/5
  Idx6/1 -> Interpolate6/2(InportIdx1), CompSup6/2, Interpolate5/3(InportIdx2), CompInfEq6/2
  Data6/1 -> Interpolate6/4(InportData1), Interpolate5/5(InportData2)
  Interpolate6/1(Out) -> Product6/1
  CompSup6/1 -> Product6/2
  CompInfEq7/1 -> Product6/3
  Product6/1 -> Sum/6
  Idx7/1 -> Interpolate7/2(InportIdx1), CompSup7/2, Interpolate6/3(InportIdx2), CompInfEq7/2
  Data7/1 -> Interpolate7/4(InportData1), Interpolate6/5(InportData2)
  Interpolate7/1(Out) -> Product7/1
  CompSup7/1 -> Product7/2
  CompInfEq8/1 -> Product7/3
  Product7/1 -> Sum/7
  Idx8/1 -> Interpolate7/3(InportIdx2), CompInfEq8/2
  Data8/1 -> Interpolate7/5(InportData2)
  Sum/1 -> Out/1

== system ap_12B_cocoSim_pp/Autopilot/Pitch_Autopilot/Altitude Mode/Rate Limiter ==
  note: Y(k)
  note: U(k)
  up : Inport
  u : Inport  Port=2
  lo : Inport  Port=3
  Constant1 : Constant  Value=Ts
  Delay Input2 : UnitDelay  Description=Store in Global RAM  DisableCoverage=on  SampleTime=-1
  Difference Inputs1 : Sum  Description=Add in CPU  DisableCoverage=on  Inputs=+-  OutDataTypeStr=Inherit: Inherit via back propagation
  Difference Inputs2 : Sum  Description=Add in CPU  OutDataTypeStr=Inherit: Inherit via back propagation
  Saturation Dynamic : simulink/Discontinuities/Saturation Dynamic  OutMin=[]  OutMax=[]  OutDataTypeStr=Inherit: Same as second input  OutDataType=fixdt(1, 16)  OutScaling=2^-10  DoSatur=off
  delta fall limit : Product  DisableCoverage=on  Inputs=**  OutDataTypeStr=Inherit: Inherit via back propagation  SaturateOnIntegerOverflow=on
  delta rise limit : Product  DisableCoverage=on  Inputs=**  OutDataTypeStr=Inherit: Inherit via back propagation  SaturateOnIntegerOverflow=on
  Y : Outport  InitialOutput=0
  wires:
  Difference Inputs1/1 -> Saturation Dynamic/2  "( U(k) - Y(k-1) )"
  u/1 -> Difference Inputs1/1
  delta fall limit/1 -> Saturation Dynamic/3
  Saturation Dynamic/1 -> Difference Inputs2/1
  Delay Input2/1 -> Difference Inputs1/2, Difference Inputs2/2  "Y(k-1)"
  Difference Inputs2/1 -> Y/1, Delay Input2/1
  up/1 -> delta rise limit/1
  delta rise limit/1 -> Saturation Dynamic/1
  lo/1 -> delta fall limit/1
  Constant1/1 -> delta rise limit/2, delta fall limit/2

== system ap_12B_cocoSim_pp/Autopilot/Pitch_Autopilot/Altitude Mode/ResetIntegratorInternal ==
  note: ic
  note: Level Reset Integration With Saturation
      | y(n) = y(n-1) + K*Ts*u(n-1)
  U : Inport
  R : Inport  Port=2
  IC : Inport  Port=3
  Constant : Constant  Value=0.2
  Constant1 : Constant  Value=Ts
  Product : Product  RndMeth=Zero
  Product1 : Product  RndMeth=Zero
  Saturation : Saturate  UpperLimit=20  LowerLimit=-20
  Sum3 : Sum
  Switch : Switch  Criteria=u2 ~= 0
  Switch1 : Switch  Criteria=u2 ~= 0
  X : UnitDelay  SampleTime=Ts
  Y : Outport
  wires:
  Product1/1 -> Sum3/1
  U/1 -> Product1/2
  Sum3/1 -> Switch1/3
  Product/1 -> Product1/1
  Switch/1 -> Saturation/1
  IC/1 -> Switch1/1, Switch/1
  Constant1/1 -> Product/2  "deltaT"
  Switch1/1 -> X/1
  Constant/1 -> Product/1  "gain"
  Saturation/1 -> Y/1, Sum3/2
  R/1 -> Switch1/2, Switch/2
  X/1 -> Switch/3

== system ap_12B_cocoSim_pp/Autopilot/Pitch_Autopilot/Basic Pitch Mode/ResetIntegratorInternal ==
  note: ic
  note: Level Reset Integration With Saturation
      | y(n) = y(n-1) + K*Ts*u(n-1)
  U : Inport
  R : Inport  Port=2
  Constant : Constant  Value=1.0
  Constant1 : Constant  Value=Ts
  Constant2 : Constant  Value=0.0
  Product : Product  RndMeth=Zero
  Product1 : Product  RndMeth=Zero
  Saturation : Saturate  UpperLimit=5  LowerLimit=-5
  Sum3 : Sum
  Switch : Switch  Criteria=u2 ~= 0
  Switch1 : Switch  Criteria=u2 ~= 0
  X : UnitDelay  SampleTime=Ts
  Y : Outport
  wires:
  Product1/1 -> Sum3/1
  U/1 -> Product1/2
  Sum3/1 -> Switch1/3
  Product/1 -> Product1/1
  Switch/1 -> Saturation/1
  Constant2/1 -> Switch1/1, Switch/1
  Constant1/1 -> Product/2  "deltaT"
  Switch1/1 -> X/1
  Constant/1 -> Product/1  "gain"
  Saturation/1 -> Y/1, Sum3/2
  R/1 -> Switch1/2, Switch/2
  X/1 -> Switch/3

== system ap_12B_cocoSim_pp/Autopilot/Pitch_Autopilot/Pitch Reference/latch ==
  note: Xold
  note: Enable
  u : Inport
  E : Inport  Port=2
  Enable : Switch  Criteria=u2 ~= 0  OutDataTypeStr=Inherit: Inherit via back propagation  ZeroCross=off
  FixPt Unit Delay1 : UnitDelay  SampleTime=Ts  HasFrameUpgradeWarning=off
  y : Outport
  wires:
  FixPt Unit Delay1/1 -> y/1, Enable/3
  Enable/1 -> FixPt Unit Delay1/1  "Xnew"
  E/1 -> Enable/2
  u/1 -> Enable/1

== system ap_12B_cocoSim_pp/Autopilot/Roll_Autopilot/Basic Roll Mode/ResetIntegratorInternal ==
  note: ic
  note: Level Reset Integration With Saturation
      | y(n) = y(n-1) + K*Ts*u(n-1)
  U : Inport
  R : Inport  Port=2
  Constant : Constant  Value=1.0
  Constant1 : Constant  Value=Ts
  Constant2 : Constant  Value=0.0
  Product : Product  RndMeth=Zero
  Product1 : Product  RndMeth=Zero
  Saturation : Saturate  UpperLimit=5  LowerLimit=-5
  Sum3 : Sum
  Switch : Switch  Criteria=u2 ~= 0
  Switch1 : Switch  Criteria=u2 ~= 0
  X : UnitDelay  SampleTime=Ts
  Y : Outport
  wires:
  Product1/1 -> Sum3/1
  U/1 -> Product1/2
  Sum3/1 -> Switch1/3
  Product/1 -> Product1/1
  Switch/1 -> Saturation/1
  Constant2/1 -> Switch1/1, Switch/1
  Constant1/1 -> Product/2  "deltaT"
  Switch1/1 -> X/1
  Constant/1 -> Product/1  "gain"
  Saturation/1 -> Y/1, Sum3/2
  R/1 -> Switch1/2, Switch/2
  X/1 -> Switch/3

== system ap_12B_cocoSim_pp/Autopilot/Roll_Autopilot/Heading Mode/angle diff ==
  plus : Inport  OutDataTypeStr=double
  minus : Inport  Port=2  OutDataTypeStr=double
  abs : Abs  ZeroCross=off
  constant : Constant  Value=180
  constant1 : Constant  Value=360
  floor : Rounding
  product : Product  RndMeth=Zero  InputSameDT=on  OutDataTypeStr=Inherit: Same as first input
  product1 : Product  Inputs=*/  RndMeth=Zero  InputSameDT=on  OutDataTypeStr=Inherit: Same as first input
  product2 : Product  RndMeth=Zero  InputSameDT=on  OutDataTypeStr=Inherit: Same as first input
  signum : Signum  ZeroCross=off
  sum : Sum  Inputs=|+-  RndMeth=Zero  InputSameDT=on  OutDataTypeStr=Inherit: Same as first input
  sum1 : Sum  Inputs=|+-  RndMeth=Zero  InputSameDT=on  OutDataTypeStr=Inherit: Same as first input
  sum2 : Sum  Inputs=|++  RndMeth=Zero  InputSameDT=on  OutDataTypeStr=Inherit: Same as first input
  diff : Outport
  wires:
  product2/1 -> product/2
  product/1 -> sum1/2
  sum2/1 -> product1/1
  constant/1 -> sum2/2
  sum1/1 -> diff/1
  signum/1 -> product/1
  floor/1 -> product2/1
  minus/1 -> sum/2
  plus/1 -> sum/1
  product1/1 -> floor/1
  sum/1 -> sum1/1, abs/1, signum/1
  abs/1 -> sum2/1
  constant1/1 -> product2/2, product1/2

== system ap_12B_cocoSim_pp/Autopilot/Roll_Autopilot/Roll Reference/latch ==
  note: Xold
  note: Enable
  u : Inport
  E : Inport  Port=2
  Enable : Switch  Criteria=u2 ~= 0  OutDataTypeStr=Inherit: Inherit via back propagation  ZeroCross=off
  FixPt Unit Delay1 : UnitDelay  SampleTime=Ts  HasFrameUpgradeWarning=off
  y : Outport
  wires:
  FixPt Unit Delay1/1 -> y/1, Enable/3
  Enable/1 -> FixPt Unit Delay1/1  "Xnew"
  E/1 -> Enable/2
  u/1 -> Enable/1

== system ap_12B_cocoSim_pp/DeHavilland Beaver Airframe/Aircraft Dynamics/6DoF (Quaternion)/3x3 CrossProduct ==
  A : Inport
  B : Inport  Port=2
  A_1 : InportShadow
  B_1 : InportShadow  Port=2
  Subsystem : aerolibutil/3x3 Cross Product/Subsystem
  Subsystem1 : aerolibutil/3x3 Cross Product/Subsystem1
  Sum : Sum  Inputs=+|-  SaturateOnIntegerOverflow=on  InputSameDT=on  OutDataTypeStr=Inherit: Same as first input
  C : Outport
  wires:
  Subsystem/1 -> Sum/1
  Subsystem1/1 -> Sum/2
  B/1 -> Subsystem/2
  A/1 -> Subsystem/1
  B_1/1 -> Subsystem1/2
  A_1/1 -> Subsystem1/1
  Sum/1 -> C/1

== system ap_12B_cocoSim_pp/DeHavilland Beaver Airframe/Aircraft Dynamics/6DoF (Quaternion)/Calculate DCM & Euler Angles ==
  p q r : Inport
  Initial Euler Angles : Constant  Value="[0    0.1303    1.9722]"
  Quaternions to  Direction Cosine Matrix : Subsystem
  Quaternions to Rotation Angles (ZYX) : Subsystem
  ResetIntegratorInternal1 : Subsystem
  Rotation Angles to Quats (ZYX) : Subsystem
  Selector : Selector  InputPortWidth=3  Indices=[3 2 1]
  Selector1 : Selector  InputPortWidth=3  Indices=[3 2 1]
  ic3 : Subsystem
  qd : Subsystem
  DCM : Outport
  Euler : Outport  Port=2
  wires:
  Selector1/1 -> Rotation Angles to Quats (ZYX)/1("R1, R2, R3")
  Selector/1 -> Euler/1
  Quaternions to Rotation Angles (ZYX)/1(R1,R2,R3) -> Selector/1
  Quaternions to  Direction Cosine Matrix/1(DCM) -> DCM/1
  p q r/1 -> qd/1(p q r)
  Initial Euler Angles/1 -> Selector1/1
  ResetIntegratorInternal1/1(Y) -> Quaternions to  Direction Cosine Matrix/1(Quat), qd/2(q0 q1 q2 q3), Quaternions to Rotation Angles (ZYX)/1(q)
  qd/1(qdot) -> ResetIntegratorInternal1/1(U)
  ic3/1(R) -> ResetIntegratorInternal1/2(R)
  ic3/2(IC) -> ResetIntegratorInternal1/3(IC)
  Rotation Angles to Quats (ZYX)/1(Quat) -> ic3/1(ic)

== system ap_12B_cocoSim_pp/DeHavilland Beaver Airframe/Aircraft Dynamics/6DoF (Quaternion)/Calculate omega_dot ==
  p q r : Inport
  "I, I_dot" : Inport  Port=2
  Moments : Inport  Port=3
  3x3 CrossProduct : Subsystem
  I x w : aerolib6dofsys/Calculate omega_dot/I x w
  I x w1 : aerolib6dofsys/Calculate omega_dot/I x w1
  Product2 : Product  Inputs=*/  Multiplication=Matrix(*)  SaturateOnIntegerOverflow=on  OutDataTypeStr=Inherit: Same as first input
  Reshape : Reshape
  Reshape1 : Reshape  OutputDimensionality=Row vector (2-D)
  Selector : Selector  NumberOfDimensions=2  InputPortWidth=2  IndexOptions=Index vector (dialog),Select all  Indices=1:3,-1
  Selector1 : Selector  NumberOfDimensions=2  InputPortWidth=2  IndexOptions=Index vector (dialog),Select all  Indices=4:6,-1
  Selector2 : Selector  NumberOfDimensions=2  InputPortWidth=2  IndexOptions=Index vector (dialog),Select all  Indices=1:3,-1
  Sum2 : Sum  Inputs=+--  SaturateOnIntegerOverflow=on
  pdot qdot rdot : Outport
  wires:
  Reshape1/1 -> Product2/1
  I x w/1 -> 3x3 CrossProduct/2(B)
  3x3 CrossProduct/1(C) -> Sum2/3
  Selector1/1 -> I x w1/1
  I x w1/1 -> Sum2/2
  Moments/1 -> Sum2/1
  Sum2/1 -> Reshape1/1
  Product2/1 -> Reshape/1
  p q r/1 -> 3x3 CrossProduct/1(A), I x w1/2, I x w/1
  "I, I_dot"/1 -> Selector2/1, Selector/1, Selector1/1
  Selector2/1 -> Product2/2
  Selector/1 -> I x w/2
  Reshape/1 -> pdot qdot rdot/1

== system ap_12B_cocoSim_pp/DeHavilland Beaver Airframe/Aircraft Dynamics/6DoF (Quaternion)/ResetIntegratorInternal ==
  note: ic
  note: Level Reset Integration With Saturation
      | y(n) = y(n-1) + K*Ts*u(n-1)
  U : Inport
  R : Inport  Port=2
  IC : Inport  Port=3
  Constant : Constant  Value=1.0
  Constant1 : Constant  Value=Ts
  Product : Product  RndMeth=Zero
  Product1 : Product  RndMeth=Zero
  Sum3 : Sum
  Switch : Switch  Criteria=u2 ~= 0
  Switch1 : Switch  Criteria=u2 ~= 0
  X : UnitDelay  SampleTime=Ts
  Y : Outport
  wires:
  Product1/1 -> Sum3/1
  U/1 -> Product1/2
  Sum3/1 -> Switch1/3
  Product/1 -> Product1/1
  IC/1 -> Switch1/1, Switch/1
  Constant1/1 -> Product/2  "deltaT"
  Switch1/1 -> X/1
  Constant/1 -> Product/1  "gain"
  Switch/1 -> Y/1, Sum3/2
  R/1 -> Switch1/2, Switch/2
  X/1 -> Switch/3

== system ap_12B_cocoSim_pp/DeHavilland Beaver Airframe/Aircraft Dynamics/6DoF (Quaternion)/ResetIntegratorInternal1 ==
  note: ic
  note: Level Reset Integration With Saturation
      | y(n) = y(n-1) + K*Ts*u(n-1)
  U : Inport
  R : Inport  Port=2
  IC : Inport  Port=3
  Constant : Constant  Value=1.0
  Constant1 : Constant  Value=Ts
  Product : Product  RndMeth=Zero
  Product1 : Product  RndMeth=Zero
  Sum3 : Sum
  Switch : Switch  Criteria=u2 ~= 0
  Switch1 : Switch  Criteria=u2 ~= 0
  X : UnitDelay  SampleTime=Ts
  Y : Outport
  wires:
  Product1/1 -> Sum3/1
  U/1 -> Product1/2
  Sum3/1 -> Switch1/3
  Product/1 -> Product1/1
  IC/1 -> Switch1/1, Switch/1
  Constant1/1 -> Product/2  "deltaT"
  Switch1/1 -> X/1
  Constant/1 -> Product/1  "gain"
  Switch/1 -> Y/1, Sum3/2
  R/1 -> Switch1/2, Switch/2
  X/1 -> Switch/3

== system ap_12B_cocoSim_pp/DeHavilland Beaver Airframe/Aircraft Dynamics/6DoF (Quaternion)/ResetIntegratorInternal2 ==
  note: Level Reset Integration With Saturation
      | y(n) = y(n-1) + K*Ts*u(n-1)
  note: ic
  U : Inport
  R : Inport  Port=2
  IC : Inport  Port=3
  Constant : Constant  Value=1.0
  Constant1 : Constant  Value=Ts
  Product : Product  RndMeth=Zero
  Product1 : Product  RndMeth=Zero
  Sum3 : Sum
  Switch : Switch  Criteria=u2 ~= 0
  Switch1 : Switch  Criteria=u2 ~= 0
  X : UnitDelay  SampleTime=Ts
  Y : Outport
  wires:
  X/1 -> Switch/3
  R/1 -> Switch/2, Switch1/2
  Constant/1 -> Product/1  "gain"
  Switch1/1 -> X/1
  Constant1/1 -> Product/2  "deltaT"
  IC/1 -> Switch/1, Switch1/1
  Product/1 -> Product1/1
  Sum3/1 -> Switch1/3
  U/1 -> Product1/2
  Product1/1 -> Sum3/1
  Switch/1 -> Sum3/2, Y/1

== system ap_12B_cocoSim_pp/DeHavilland Beaver Airframe/Aircraft Dynamics/6DoF (Quaternion)/Subsystem ==
  Vb : Inport
  forces : Inport  Port=2
  "mass " : Inport  Port=3
  m_dot : Inport  Port=4  OutDataTypeStr=double
  I : Inport  Port=5  OutDataTypeStr=double
  I_dot : Inport  Port=6  OutDataTypeStr=double
  Constant : Constant  Value=beaver_mass  OutDataTypeStr=Inherit: Inherit via back propagation
  Constant1 : Constant  Value=[inertia; zeros(3,3)]  OutDataTypeStr=Inherit: Inherit via back propagation
  Ground : Ground
  Terminator{,1..4} (5 alike) : Terminator
  "forces " : Outport
  mass : Outport  Port=2
  "inertia, 0" : Outport  Port=3
  Out9 : Outport  Port=4
  wires:
  Constant1/1 -> "inertia, 0"/1
  "mass "/1 -> Terminator3/1
  forces/1 -> "forces "/1
  Vb/1 -> Terminator4/1
  Constant/1 -> mass/1
  I_dot/1 -> Terminator2/1
  I/1 -> Terminator/1
  Ground/1 -> Out9/1
  m_dot/1 -> Terminator1/1

== system ap_12B_cocoSim_pp/DeHavilland Beaver Airframe/Aircraft Dynamics/6DoF (Quaternion)/ic1 ==
  Constant : Constant  Value=0
  Constant1 : Constant  Value=xme_0
  Unit Delay : UnitDelay  InitialCondition=1  SampleTime=-1
  R : Outport
  IC : Outport  Port=2
  wires:
  Constant/1 -> Unit Delay/1
  Unit Delay/1 -> R/1
  Constant1/1 -> IC/1

== system ap_12B_cocoSim_pp/DeHavilland Beaver Airframe/Aircraft Dynamics/6DoF (Quaternion)/ic2 ==
  Constant : Constant  Value=0
  Constant1 : Constant  Value=[44.54;2.714;5.836]
  Unit Delay : UnitDelay  InitialCondition=1  SampleTime=-1
  R : Outport
  IC : Outport  Port=2
  wires:
  Constant1/1 -> IC/1
  Constant/1 -> Unit Delay/1
  Unit Delay/1 -> R/1

== system ap_12B_cocoSim_pp/DeHavilland Beaver Airframe/Aircraft Dynamics/6DoF (Quaternion)/ic3 ==
  Constant : Constant  Value=0
  Constant1 : Constant  Value=0
  Unit Delay : UnitDelay  InitialCondition=1  SampleTime=-1
  R : Outport
  IC : Outport  Port=2
  wires:
  Constant/1 -> Unit Delay/1
  Unit Delay/1 -> R/1
  Constant1/1 -> IC/1

== system ap_12B_cocoSim_pp/DeHavilland Beaver Airframe/Aircraft Dynamics/Total Forces  and Moments/Actuators ==
  Pilot : Inport
  Bus Selector2 : BusSelector  OutputSignals=uaero
  Demux : Demux
  Initial inputs for aero : Constant  Value=uaero0
  Mux : Mux
  Scope : Scope
      settings: SaveName=ScopeData13
  Sum1 : Sum  Inputs=++|  SaturateOnIntegerOverflow=on  InputSameDT=on  OutDataTypeStr=Inherit: Same as first input
  sof : Subsystem
  sof1 : Subsystem
  sof2 : Subsystem
  uaero-out : Outport
  wires:
  Pilot/1 -> Bus Selector2/1
  Initial inputs for aero/1 -> Sum1/1
  Demux/4 -> Mux/4
  Demux/1 -> sof/1(Ac_dem)
  Demux/2 -> sof1/1(Ac_dem)
  Sum1/1 -> Demux/1
  sof/1(Ac_ac) -> Mux/1
  sof1/1(Ac_ac) -> Mux/2
  Bus Selector2/1 -> Sum1/2  "<uaero>"
  Mux/1 -> Scope/1, uaero-out/1
  Demux/3 -> sof2/1(Ac_dem)
  sof2/1(Ac_ac) -> Mux/3

== system ap_12B_cocoSim_pp/DeHavilland Beaver Airframe/Aircraft Dynamics/Total Forces  and Moments/Aerodynamics ==
  Uaero : Inport
  FltParams : Inport  Port=2
  Actuator Increments : Subsystem
  Body Rate Damping : Subsystem
  Bus Selector1 : BusSelector  OutputSignals=alpha,beta
  Bus Selector2 : BusSelector  OutputSignals=V,pqr_tot
  Datum Coefficients : Subsystem
  Sum1 : Sum  Inputs=|++  SaturateOnIntegerOverflow=on
  Sum4 : Sum  Inputs=|++  SaturateOnIntegerOverflow=on
  Aero Coefficients : Outport
  wires:
  Bus Selector1/2 -> Actuator Increments/2(beta), Datum Coefficients/2(beta)  "<beta>"
  Bus Selector2/1 -> Body Rate Damping/1(V)  "<V>"
  Bus Selector2/2 -> Body Rate Damping/2(p,q,r)  "<pqr_tot>"
  Uaero/1 -> Actuator Increments/3(Actuator Deflections)
  Bus Selector1/1 -> Actuator Increments/1(alpha), Datum Coefficients/1(alpha)  "<alpha>"
  FltParams/1 -> Bus Selector1/1, Bus Selector2/1
  Datum Coefficients/1(Coefficients) -> Sum4/1
  Actuator Increments/1(Coefficients) -> Sum4/2
  Sum4/1 -> Sum1/1
  Body Rate Damping/1(Coefficients) -> Sum1/2
  Sum1/1 -> Aero Coefficients/1

== system ap_12B_cocoSim_pp/DeHavilland Beaver Airframe/Aircraft Dynamics/Total Forces  and Moments/Engine  ==
  Fltparams : Inport
  Pilot : Inport  Port=2
  rho : Inport  Port=3
  Bus Selector4 : BusSelector  OutputSignals=V,alpha
  eng : Subsystem
  pow : Subsystem
  Engine Coefficients : Outport
  wires:
  Bus Selector4/1 -> pow/3(V)  "<V>"
  rho/1 -> pow/1(rho)
  Bus Selector4/2 -> eng/2(alpha)  "<alpha>"
  eng/1(Cprop) -> Engine Coefficients/1
  Pilot/1 -> pow/2(Pilot)
  pow/1(dpt) -> eng/1(dpt)
  Fltparams/1 -> Bus Selector4/1

== system ap_12B_cocoSim_pp/DeHavilland Beaver Airframe/Aircraft Dynamics/Total Forces  and Moments/Forces and Moments ==
  Aero Coefficients : Inport
  Fltparams : Inport  Port=2
  Engine Coefficients : Inport  Port=3
  Aero F&M : Subsystem
  Bus Selector4 : BusSelector  OutputSignals=Qdyn
  Scope : Scope
      settings: SaveName=ScopeData22
  Sum : Sum  Inputs=++|  SaturateOnIntegerOverflow=on  InputSameDT=on  OutDataTypeStr=Inherit: Same as first input
  neglect center of gravity  and center of pressure effects : Constant  Value=[0 0 0]
  XYZ : Outport
  LMN : Outport  Port=2
  wires:
  Sum/1 -> Aero F&M/1(Coefficients)
  Aero Coefficients/1 -> Sum/2
  Engine Coefficients/1 -> Sum/1
  Fltparams/1 -> Bus Selector4/1
  Aero F&M/1(Forces) -> XYZ/1
  neglect center of gravity  and center of pressure effects/1 -> Aero F&M/4(CP), Aero F&M/3(CG)
  Bus Selector4/1 -> Scope/1, Aero F&M/2(qbar)  "<Qdyn>"
  Aero F&M/2(Moments) -> LMN/1

== system ap_12B_cocoSim_pp/DeHavilland Beaver Airframe/Aircraft Dynamics/Total Forces  and Moments/Gravity  ==
  g : Inport
  DCM : Inport  Port=2
  Constant : Constant  Value=0.0
  Gain : Gain  Gain=beaver_mass
  Inertial to Body : Product  Multiplication=Matrix(*)  SaturateOnIntegerOverflow=on  InputSameDT=on  OutDataTypeStr=Inherit: Same as first input
  Mux : Mux  Inputs=3
  Reshape1 : Reshape
  Fgrav : Outport
  wires:
  Inertial to Body/1 -> Reshape1/1
  g/1 -> Gain/1
  DCM/1 -> Inertial to Body/1
  Mux/1 -> Inertial to Body/2
  Reshape1/1 -> Fgrav/1
  Constant/1 -> Mux/2, Mux/1
  Gain/1 -> Mux/3

== system ap_12B_cocoSim_pp/Autopilot/Pitch_Autopilot/Altitude Mode/Lookup Table_pp/Interpolate1 ==
  InportIn : Inport
  InportIdx1 : Inport  Port=2
  InportIdx2 : Inport  Port=3
  InportData1 : Inport  Port=4
  InportData2 : Inport  Port=5
  Interpolate : Product  Inputs=*/*  SaturateOnIntegerOverflow=on  RndMeth=Zero  InputSameDT=on  OutDataTypeStr=Inherit: Same as first input
  Sum1 : Sum  Inputs=+-  SaturateOnIntegerOverflow=on  InputSameDT=on  OutDataTypeStr=Inherit: Same as first input
  Sum2 : Sum  Inputs=-+  SaturateOnIntegerOverflow=on  InputSameDT=on  OutDataTypeStr=Inherit: Same as first input
  Sum3 : Sum  Inputs=-+  SaturateOnIntegerOverflow=on  InputSameDT=on  OutDataTypeStr=Inherit: Same as first input
  Sum4 : Sum  SaturateOnIntegerOverflow=on  InputSameDT=on  OutDataTypeStr=Inherit: Same as first input
  Out : Outport
  wires:
  InportIn/1 -> Sum1/1
  InportIdx1/1 -> Sum1/2, Sum2/1
  InportIdx2/1 -> Sum2/2
  InportData1/1 -> Sum3/1, Sum4/2
  InportData2/1 -> Sum3/2
  Sum1/1 -> Interpolate/1
  Sum2/1 -> Interpolate/2
  Sum3/1 -> Interpolate/3
  Interpolate/1 -> Sum4/1
  Sum4/1 -> Out/1

== system ap_12B_cocoSim_pp/Autopilot/Pitch_Autopilot/Altitude Mode/Lookup Table_pp/Interpolate2 ==
  InportIn : Inport
  InportIdx1 : Inport  Port=2
  InportIdx2 : Inport  Port=3
  InportData1 : Inport  Port=4
  InportData2 : Inport  Port=5
  Interpolate : Product  Inputs=*/*  SaturateOnIntegerOverflow=on  RndMeth=Zero  InputSameDT=on  OutDataTypeStr=Inherit: Same as first input
  Sum1 : Sum  Inputs=+-  SaturateOnIntegerOverflow=on  InputSameDT=on  OutDataTypeStr=Inherit: Same as first input
  Sum2 : Sum  Inputs=-+  SaturateOnIntegerOverflow=on  InputSameDT=on  OutDataTypeStr=Inherit: Same as first input
  Sum3 : Sum  Inputs=-+  SaturateOnIntegerOverflow=on  InputSameDT=on  OutDataTypeStr=Inherit: Same as first input
  Sum4 : Sum  SaturateOnIntegerOverflow=on  InputSameDT=on  OutDataTypeStr=Inherit: Same as first input
  Out : Outport
  wires:
  InportIn/1 -> Sum1/1
  InportIdx1/1 -> Sum1/2, Sum2/1
  InportIdx2/1 -> Sum2/2
  InportData1/1 -> Sum3/1, Sum4/2
  InportData2/1 -> Sum3/2
  Sum1/1 -> Interpolate/1
  Sum2/1 -> Interpolate/2
  Sum3/1 -> Interpolate/3
  Interpolate/1 -> Sum4/1
  Sum4/1 -> Out/1

== system ap_12B_cocoSim_pp/Autopilot/Pitch_Autopilot/Altitude Mode/Lookup Table_pp/Interpolate3 ==
  InportIn : Inport
  InportIdx1 : Inport  Port=2
  InportIdx2 : Inport  Port=3
  InportData1 : Inport  Port=4
  InportData2 : Inport  Port=5
  Interpolate : Product  Inputs=*/*  SaturateOnIntegerOverflow=on  RndMeth=Zero  InputSameDT=on  OutDataTypeStr=Inherit: Same as first input
  Sum1 : Sum  Inputs=+-  SaturateOnIntegerOverflow=on  InputSameDT=on  OutDataTypeStr=Inherit: Same as first input
  Sum2 : Sum  Inputs=-+  SaturateOnIntegerOverflow=on  InputSameDT=on  OutDataTypeStr=Inherit: Same as first input
  Sum3 : Sum  Inputs=-+  SaturateOnIntegerOverflow=on  InputSameDT=on  OutDataTypeStr=Inherit: Same as first input
  Sum4 : Sum  SaturateOnIntegerOverflow=on  InputSameDT=on  OutDataTypeStr=Inherit: Same as first input
  Out : Outport
  wires:
  InportIn/1 -> Sum1/1
  InportIdx1/1 -> Sum1/2, Sum2/1
  InportIdx2/1 -> Sum2/2
  InportData1/1 -> Sum3/1, Sum4/2
  InportData2/1 -> Sum3/2
  Sum1/1 -> Interpolate/1
  Sum2/1 -> Interpolate/2
  Sum3/1 -> Interpolate/3
  Interpolate/1 -> Sum4/1
  Sum4/1 -> Out/1

== system ap_12B_cocoSim_pp/Autopilot/Pitch_Autopilot/Altitude Mode/Lookup Table_pp/Interpolate4 ==
  InportIn : Inport
  InportIdx1 : Inport  Port=2
  InportIdx2 : Inport  Port=3
  InportData1 : Inport  Port=4
  InportData2 : Inport  Port=5
  Interpolate : Product  Inputs=*/*  SaturateOnIntegerOverflow=on  RndMeth=Zero  InputSameDT=on  OutDataTypeStr=Inherit: Same as first input
  Sum1 : Sum  Inputs=+-  SaturateOnIntegerOverflow=on  InputSameDT=on  OutDataTypeStr=Inherit: Same as first input
  Sum2 : Sum  Inputs=-+  SaturateOnIntegerOverflow=on  InputSameDT=on  OutDataTypeStr=Inherit: Same as first input
  Sum3 : Sum  Inputs=-+  SaturateOnIntegerOverflow=on  InputSameDT=on  OutDataTypeStr=Inherit: Same as first input
  Sum4 : Sum  SaturateOnIntegerOverflow=on  InputSameDT=on  OutDataTypeStr=Inherit: Same as first input
  Out : Outport
  wires:
  InportIn/1 -> Sum1/1
  InportIdx1/1 -> Sum1/2, Sum2/1
  InportIdx2/1 -> Sum2/2
  InportData1/1 -> Sum3/1, Sum4/2
  InportData2/1 -> Sum3/2
  Sum1/1 -> Interpolate/1
  Sum2/1 -> Interpolate/2
  Sum3/1 -> Interpolate/3
  Interpolate/1 -> Sum4/1
  Sum4/1 -> Out/1
